simulink library "Nav_sys_org"  (R2018b)
settings: Solver=VariableStepAuto  StartTime=0.0  StopTime=10.0  RelTol=1e-3
libraries: simulink x2
settings Model: Creator=Andrew Garcia  LastModifiedBy=Andrew Garcia

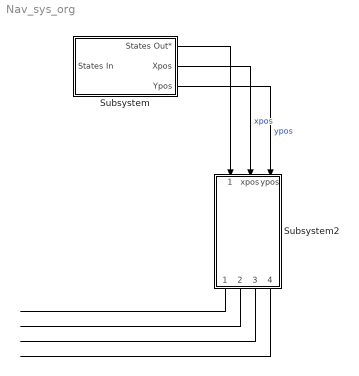
== system Nav_sys_org ==
  Subsystem : Subsystem
  Subsystem2 : Subsystem
  wires:
  Subsystem2/4(Heading/Yaw) -> ?
  Subsystem2/3(Zpos) -> ?
  Subsystem2/2(Ypos) -> ?
  Subsystem2/1(Xpos) -> ?
  Subsystem/3(Ypos) -> Subsystem2/3(ypos)  "ypos"
  Subsystem/2(Xpos) -> Subsystem2/2(xpos)  "xpos"
  Subsystem/1(States Out*) -> Subsystem2/1(States In*)
  ? -> Subsystem/1(States In)

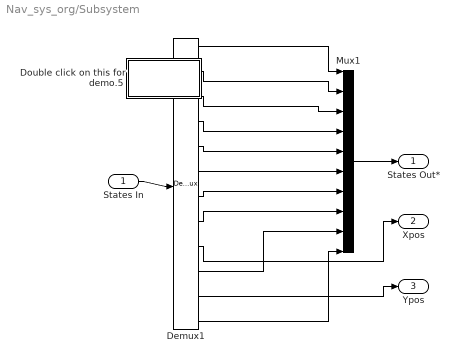
== system Nav_sys_org/Subsystem ==
  States In : Inport
  Demux1 : Demux  Outputs=12
  Double click on this for demo.5 : Subsystem
      settings: OpenFcn=optsiminit
      mask Display: disp('optsiminit')
  Mux1 : Mux  Inputs=10
  States Out* : Outport
  Xpos : Outport  Port=2
  Ypos : Outport  Port=3
  wires:
  States In/1 -> Demux1/1
  Demux1/11 -> Ypos/1
  Demux1/9 -> Xpos/1
  Mux1/1 -> States Out*/1
  Demux1/12 -> Mux1/10
  Demux1/10 -> Mux1/9
  Demux1/8 -> Mux1/8
  Demux1/7 -> Mux1/7
  Demux1/6 -> Mux1/6
  Demux1/5 -> Mux1/5
  Demux1/4 -> Mux1/4
  Demux1/3 -> Mux1/3
  Demux1/2 -> Mux1/2
  Demux1/1 -> Mux1/1

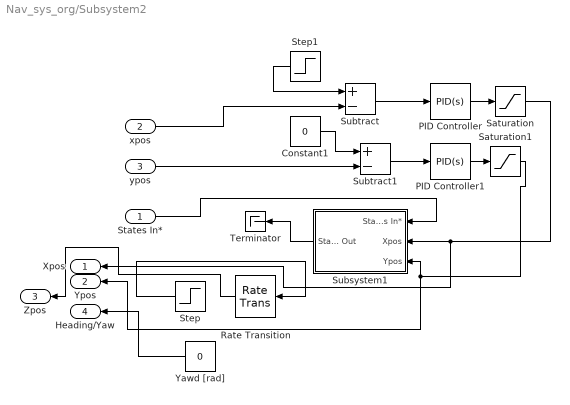
== system Nav_sys_org/Subsystem2 ==
  States In* : Inport
  xpos : Inport  Port=2
  ypos : Inport  Port=3
  Constant1 : Constant  Value=0
  PID Controller : simulink/Continuous/PID Controller  Controller=PID  Form=Parallel  TimeDomain=Continuous-time  SampleTime=-1  IntegratorMethod=Forward Euler  FilterMethod=Forward Euler  ControllerParametersSource=internal  P=0.8  I=0.2  D=0  UseFilter=on  N=100  TunerSelectOption=Transfer Function Based (PID Tuner App)  InitialConditionSource=internal  InitialConditionForIntegrator=0  InitialConditionForFilter=0  DifferentiatorICPrevScaledInput=0  ExternalReset=none  TrackingMode=off  Kt=1  LimitOutput=off  UpperSaturationLimit=inf  LowerSaturationLimit=-inf  LinearizeAsGain=off  AntiWindupMode=none  Kb=1  POutMin=[]  POutMax=[]  IOutMin=[]  IOutMax=[]  DOutMin=[]  DOutMax=[]  NOutMin=[]  NOutMax=[]  SumOutMin=[]  SumOutMax=[]  SaturationOutMin=[]  SaturationOutMax=[]  PParamMin=[]  PParamMax=[]  IParamMin=[]  IParamMax=[]  DParamMin=[]  DParamMax=[]  NParamMin=[]  NParamMax=[]  KbParamMin=[]  KbParamMax=[]  KtParamMin=[]  KtParamMax=[]  KbOutMin=[]  KbOutMax=[]  KtOutMin=[]  KtOutMax=[]  IntegratorOutMin=[]  IntegratorOutMax=[]  FilterOutMin=[]  FilterOutMax=[]  SumI1OutMin=[]  SumI1OutMax=[]  SumI2OutMin=[]  SumI2OutMax=[]  SumI3OutMin=[]  SumI3OutMax=[]  SumI4OutMin=[]  SumI4OutMax=[]  SumDOutMin=[]  SumDOutMax=[]  DifferentiatorOutMin=[]  DifferentiatorOutMax=[]  FilterDiffOutCoefMin=[]  FilterDiffOutCoefMax=[]  ReciprocalOutMin=[]  ReciprocalOutMax=[]  SumDenOutMin=[]  SumDenOutMax=[]  SumNumOutMin=[]  SumNumOutMax=[]  DivideOutMin=[]  DivideOutMax=[]  IntegratorContinuousStateAttributes=''  IntegratorStateMustResolveToSignalObject=off  IntegratorRTWStateStorageClass=Auto  FilterContinuousStateAttributes=''  FilterStateMustResolveToSignalObject=off  FilterRTWStateStorageClass=Auto  ParallelPVariant=InternalParameters  IdealPVariant=Disabled  IVariant=InternalParameters  DVariant=InternalParameters  IntegratorVariant=Continuous  SatVariant=Disabled  AWVariant=Passthrough  PCopyVariant=Disabled  TRVariant=Disabled  FdbkBlocksVariant=Forward  IdealPFdbkVariant=Disabled  SatFdbkVariant=Disabled  DerivativeFilterVariant=ContFilter  NVariant=InternalParameters  NCopyVariant=Disabled  FilterICVariant=InternalICsFilter  IntegratorICVariant=InternalICs  ExternalResetVariant=Disabled  TRSumVariant=Passthrough  SumFdbkVariant=Disabled  SumVariant=Sum_PID
  PID Controller1 : simulink/Continuous/PID Controller  Controller=PID  Form=Parallel  TimeDomain=Continuous-time  SampleTime=-1  IntegratorMethod=Forward Euler  FilterMethod=Forward Euler  ControllerParametersSource=internal  P=1  I=0.2  D=0  UseFilter=on  N=100  TunerSelectOption=Transfer Function Based (PID Tuner App)  InitialConditionSource=internal  InitialConditionForIntegrator=0  InitialConditionForFilter=0  DifferentiatorICPrevScaledInput=0  ExternalReset=none  TrackingMode=off  Kt=1  LimitOutput=off  UpperSaturationLimit=inf  LowerSaturationLimit=-inf  LinearizeAsGain=off  AntiWindupMode=none  Kb=1  POutMin=[]  POutMax=[]  IOutMin=[]  IOutMax=[]  DOutMin=[]  DOutMax=[]  NOutMin=[]  NOutMax=[]  SumOutMin=[]  SumOutMax=[]  SaturationOutMin=[]  SaturationOutMax=[]  PParamMin=[]  PParamMax=[]  IParamMin=[]  IParamMax=[]  DParamMin=[]  DParamMax=[]  NParamMin=[]  NParamMax=[]  KbParamMin=[]  KbParamMax=[]  KtParamMin=[]  KtParamMax=[]  KbOutMin=[]  KbOutMax=[]  KtOutMin=[]  KtOutMax=[]  IntegratorOutMin=[]  IntegratorOutMax=[]  FilterOutMin=[]  FilterOutMax=[]  SumI1OutMin=[]  SumI1OutMax=[]  SumI2OutMin=[]  SumI2OutMax=[]  SumI3OutMin=[]  SumI3OutMax=[]  SumI4OutMin=[]  SumI4OutMax=[]  SumDOutMin=[]  SumDOutMax=[]  DifferentiatorOutMin=[]  DifferentiatorOutMax=[]  FilterDiffOutCoefMin=[]  FilterDiffOutCoefMax=[]  ReciprocalOutMin=[]  ReciprocalOutMax=[]  SumDenOutMin=[]  SumDenOutMax=[]  SumNumOutMin=[]  SumNumOutMax=[]  DivideOutMin=[]  DivideOutMax=[]  IntegratorContinuousStateAttributes=''  IntegratorStateMustResolveToSignalObject=off  IntegratorRTWStateStorageClass=Auto  FilterContinuousStateAttributes=''  FilterStateMustResolveToSignalObject=off  FilterRTWStateStorageClass=Auto  ParallelPVariant=InternalParameters  IdealPVariant=Disabled  IVariant=InternalParameters  DVariant=InternalParameters  IntegratorVariant=Continuous  SatVariant=Disabled  AWVariant=Passthrough  PCopyVariant=Disabled  TRVariant=Disabled  FdbkBlocksVariant=Forward  IdealPFdbkVariant=Disabled  SatFdbkVariant=Disabled  DerivativeFilterVariant=ContFilter  NVariant=InternalParameters  NCopyVariant=Disabled  FilterICVariant=InternalICsFilter  IntegratorICVariant=InternalICs  ExternalResetVariant=Disabled  TRSumVariant=Passthrough  SumFdbkVariant=Disabled  SumVariant=Sum_PID
  Rate Transition : RateTransition
  Saturation : Saturate  UpperLimit=20  LowerLimit=-20
  Saturation1 : Saturate  UpperLimit=20  LowerLimit=-20
  Step : Step  Time=10  After=0  SampleTime=0
  Step1 : Step  Time=5  After=0  SampleTime=0
  Subsystem1 : Subsystem
  Subtract : Sum  Inputs=+-
  Subtract1 : Sum  Inputs=+-
  Terminator : Terminator
  Yawd [rad] : Constant  Value=0
  Xpos : Outport
  Ypos : Outport  Port=2
  Zpos : Outport  Port=3
  Heading/Yaw : Outport  Port=4
  wires:
  Yawd [rad]/1 -> Heading/Yaw/1
  xpos/1 -> Subtract/2
  States In*/1 -> Subsystem1/1(States In*)
  Step1/1 -> Subtract/1
  PID Controller/1 -> Saturation/1
  Subsystem1/1(States Out) -> Terminator/1
  ypos/1 -> Subtract1/2
  PID Controller1/1 -> Saturation1/1
  Subtract1/1 -> PID Controller1/1
  Subtract/1 -> PID Controller/1
  Rate Transition/1 -> Zpos/1
  Step/1 -> Rate Transition/1
  Constant1/1 -> Subtract1/1
  Saturation1/1 -> Ypos/1, Subsystem1/3(Ypos)
  Saturation/1 -> Subsystem1/2(Xpos), Xpos/1

== system Nav_sys_org/Subsystem/Double click on this for demo.5 ==

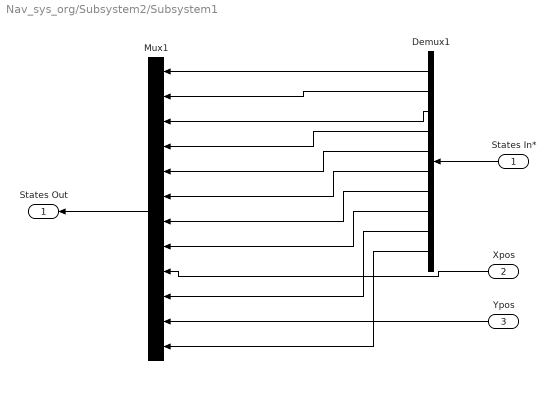
== system Nav_sys_org/Subsystem2/Subsystem1 ==
  States In* : Inport
  Xpos : Inport  Port=2
  Ypos : Inport  Port=3
  Demux1 : Demux  Outputs=10
  Mux1 : Mux  Inputs=12
  States Out : Outport
  wires:
  Mux1/1 -> States Out/1
  Ypos/1 -> Mux1/11
  Xpos/1 -> Mux1/9
  Demux1/9 -> Mux1/10
  Demux1/10 -> Mux1/12
  Demux1/8 -> Mux1/8
  Demux1/7 -> Mux1/7
  Demux1/6 -> Mux1/6
  Demux1/5 -> Mux1/5
  Demux1/4 -> Mux1/4
  Demux1/3 -> Mux1/3
  Demux1/2 -> Mux1/2
  Demux1/1 -> Mux1/1
  States In*/1 -> Demux1/1
